simulink library "bcm"  (R2021b)
settings: Solver=VariableStepAuto  StartTime=0.0  StopTime=10.0  RelTol=1e-3
undefined symbols (not defined in the file or in its folder): KBCM_BSDFlashOFFT_cnt, KBCM_BSDFlashONT_cnt, KBCM_BSDRedMode_enum, KBCM_BSDWarnReqLv_enum, KBCM_FireBuzzerEN_flg, KBCM_FLTurnLPLv_A, KBCM_FRTurnLPLv_A, KBCM_LampOFFV_V, KBCM_LampONV_V, KBCM_LightDelayOFFT_Cnt, KBCM_LightDelayONT_Cnt, KBCM_RLTurnLPLv_A, KBCM_RRTurnLPLv_A
libraries: simulink x103, hdlsllib x1
(part 3 of 3)

== system bcm/BCM/Subsystem/Subsystem/Subsystem ==
  In1 : Inport
  Add : Sum  Inputs=-+
  Compare To Constant : simulink/Logic and Bit Operations/Compare To Constant  relop=>  const=0  OutDataTypeStr=boolean
  Constant : Constant  Value=500
  Constant1 : Constant
  Constant2 : Constant  Value=0
  Data Type Conversion{,1..3} (4 alike) : DataTypeConversion  OutDataTypeStr=uint16
  Detect Increase : simulink/Logic and Bit Operations/Detect Increase  vinit=0.0  OutDataTypeStr=boolean
  Switch : Switch  Criteria=u2 > Threshold
  Switch1 : Switch  Criteria=u2 > Threshold
  Unit Delay : UnitDelay  SampleTime=-1  HasFrameUpgradeWarning=on
  Out1 : Outport
  wires:
  Detect Increase/1 -> Switch/2
  In1/1 -> Detect Increase/1
  Constant/1 -> Data Type Conversion/1
  Data Type Conversion/1 -> Switch/1
  Switch/1 -> Data Type Conversion1/1
  Add/1 -> Switch/3
  Switch1/1 -> Add/1
  Unit Delay/1 -> Switch1/2, Add/2
  Constant1/1 -> Data Type Conversion2/1
  Data Type Conversion2/1 -> Switch1/1
  Data Type Conversion3/1 -> Switch1/3
  Constant2/1 -> Data Type Conversion3/1
  Data Type Conversion1/1 -> Compare To Constant/1, Unit Delay/1
  Compare To Constant/1 -> Out1/1

== system bcm/BCM/Subsystem/Subsystem/Subsystem1 ==
  In1 : Inport
  Add : Sum  Inputs=-+
  Compare To Constant : simulink/Logic and Bit Operations/Compare To Constant  relop=>  const=0  OutDataTypeStr=boolean
  Constant : Constant  Value=500
  Constant1 : Constant
  Constant2 : Constant  Value=0
  Data Type Conversion{,1..3} (4 alike) : DataTypeConversion  OutDataTypeStr=uint16
  Detect Increase : simulink/Logic and Bit Operations/Detect Increase  vinit=0.0  OutDataTypeStr=boolean
  Switch : Switch  Criteria=u2 > Threshold
  Switch1 : Switch  Criteria=u2 > Threshold
  Unit Delay : UnitDelay  SampleTime=-1  HasFrameUpgradeWarning=on
  Out1 : Outport
  wires:
  Compare To Constant/1 -> Out1/1
  Data Type Conversion1/1 -> Unit Delay/1, Compare To Constant/1
  Constant2/1 -> Data Type Conversion3/1
  Data Type Conversion3/1 -> Switch1/3
  Data Type Conversion2/1 -> Switch1/1
  Constant1/1 -> Data Type Conversion2/1
  Unit Delay/1 -> Add/2, Switch1/2
  Switch1/1 -> Add/1
  Add/1 -> Switch/3
  Switch/1 -> Data Type Conversion1/1
  Data Type Conversion/1 -> Switch/1
  Constant/1 -> Data Type Conversion/1
  In1/1 -> Detect Increase/1
  Detect Increase/1 -> Switch/2

== system bcm/BCM/Subsystem/ExteriorLight/Subsystem4/DelayOFF ==
  note: 6 sec
  Low : Inport
  Add : Sum
  Constant4 : Constant  Value=0
  Constant5 : Constant  Value=KBCM_LightDelayOFFT_Cnt
  Data Type Conversion2 : DataTypeConversion  OutDataTypeStr=uint16
  Data Type Conversion3 : DataTypeConversion  OutDataTypeStr=uint16
  Relational Operator2 : RelationalOperator  Operator=<  OutDataTypeStr=boolean  RndMeth=Simplest
  Switch1 : Switch  Criteria=u2 > Threshold
  Unit Delay1 : UnitDelay  SampleTime=-1  HasFrameUpgradeWarning=on
  DelayOFF : Outport
  wires:
  Add/1 -> Switch1/3
  Data Type Conversion2/1 -> Switch1/1
  Unit Delay1/1 -> Relational Operator2/1, Add/1
  Constant4/1 -> Data Type Conversion2/1
  Constant5/1 -> Relational Operator2/2
  Switch1/1 -> Unit Delay1/1
  Data Type Conversion3/1 -> Add/2
  Low/1 -> Switch1/2
  Relational Operator2/1 -> DelayOFF/1, Data Type Conversion3/1

== system bcm/BCM/Subsystem/ExteriorLight/Subsystem4/DelayON ==
  note: 0.5 sec
  High : Inport
  Add : Sum
  Constant4 : Constant  Value=0
  Constant5 : Constant  Value=KBCM_LightDelayONT_Cnt
  Data Type Conversion2 : DataTypeConversion  OutDataTypeStr=uint16
  Data Type Conversion3 : DataTypeConversion  OutDataTypeStr=uint16
  Logical Operator : Logic  Operator=NOT  AllPortsSameDT=off  OutDataTypeStr=boolean
  Relational Operator2 : RelationalOperator  Operator=<  OutDataTypeStr=boolean  RndMeth=Simplest
  Switch1 : Switch  Criteria=u2 > Threshold
  Unit Delay1 : UnitDelay  SampleTime=-1  HasFrameUpgradeWarning=on
  DelayON : Outport
  wires:
  High/1 -> Switch1/2
  Data Type Conversion3/1 -> Add/2
  Relational Operator2/1 -> Logical Operator/1, Data Type Conversion3/1
  Switch1/1 -> Unit Delay1/1
  Constant5/1 -> Relational Operator2/2
  Constant4/1 -> Data Type Conversion2/1
  Unit Delay1/1 -> Add/1, Relational Operator2/1
  Data Type Conversion2/1 -> Switch1/3
  Add/1 -> Switch1/1
  Logical Operator/1 -> DelayON/1
